simulink model "LedLogic"  (R2023a)
settings: Solver=VariableStepAuto  StartTime=0.0  StopTime=1  RelTol=1e-3
libraries: simulink x1
settings Model: Creator=ptl7263  LastModifiedBy=ptl7263

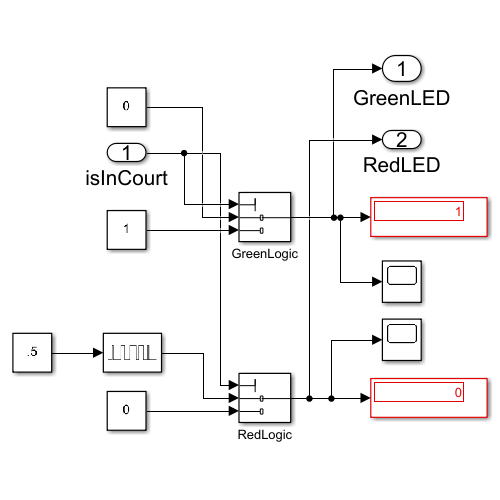
[thumbnail: Simulink's stored preview of the top-level diagram]
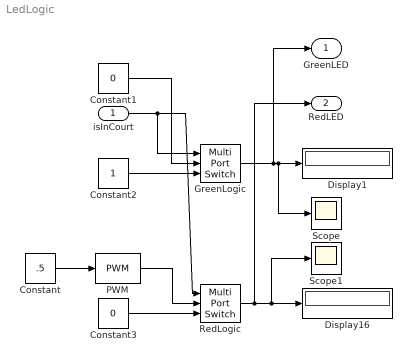
== system LedLogic ==
  isInCourt : Inport  OutDataTypeStr=boolean
  Constant : Constant  Value=.5
  Constant1 : Constant  Value=0
  Constant2 : Constant
  Constant3 : Constant  Value=0
  Display1 : Display
  Display16 : Display
  GreenLogic : MultiPortSwitch  DataPortOrder=Zero-based contiguous  Inputs=2  zeroidx=on  SaturateOnIntegerOverflow=off  InputSameDT=off
  PWM : simulink/Discontinuities/PWM  DisableCoverage=on  Period=.1  InitialDelay=0  DisallowZeroDutyCycle=off  RunAtFixedTimeIntervals=off  SampleTime=0.1
  RedLogic : MultiPortSwitch  DataPortOrder=Zero-based contiguous  Inputs=2  zeroidx=on  SaturateOnIntegerOverflow=off  InputSameDT=off
  Scope : Scope
  Scope1 : Scope
  GreenLED : Outport  VectorParamsAs1DForOutWhenUnconnected=off
  RedLED : Outport  Port=2  VectorParamsAs1DForOutWhenUnconnected=off
  wires:
  GreenLogic/1 -> Scope/1, Display1/1, GreenLED/1
  Constant/1 -> PWM/1
  isInCourt/1 -> RedLogic/1, GreenLogic/1
  Constant1/1 -> GreenLogic/2
  Constant3/1 -> RedLogic/3
  Constant2/1 -> GreenLogic/3
  PWM/1 -> RedLogic/2
  RedLogic/1 -> Scope1/1, Display16/1, RedLED/1
